simulink model "ai_optimal_path_v1"  (R2019a)
settings: Solver=FixedStepDiscrete  StartTime=0.0  StopTime=inf  FixedStep=0.2  RelTol=1e-3  EnableMultiTasking=on
undefined symbols (not defined in the file): Data, Data_SL_Info
libraries: robotlib x15
(part 1 of 2)
settings Model: Creator=USER  LastModifiedBy=USER
settings SolverCC: InsertRTBMode=Never (minimum delay)
settings DataIOCC: ReturnWorkspaceOutputs=off
settings OptimizationCC: StrengthReduction=on  PassReuseOutputArgsAs=Individual arguments  MaxStackSize=64  OptimizeBlockOrder=speed  OptimizationPriority=Speed  OptimizationCustomize=off  MultiThreadedLoops=on
settings DebuggingCC: ParameterTunabilityLossMsg=error  PregeneratedLibrarySubsystemCodeDiagnostic=none  ArithmeticOperatorsInVariantConditions=warning
settings HardwareCC: ProdBitPerPointer=32  ProdBitPerSizeT=32  ProdBitPerPtrDiffT=32  ProdLargestAtomicFloat=None  ProdIntDivRoundTo=Undefined  ProdEndianess=Unspecified  ProdWordSize=32  ProdHWDeviceType=Generic->Unspecified (assume 32-bit Generic)
settings SFSimCC: SimUseLocalCustomCode=off  MATLABDynamicMemAlloc=off
settings RTWCC: SystemTargetFile=ert.tlc  HardwareBoard=Robot Operating System (ROS)  TLCOptions="-aInlineSetEventsForThisBaseRateFcn=TLC_FALSE -aSuppressMultiTaskScheduler=TLC_FALSE  -aRateBasedStepFcn=0"  TemplateMakefile=ert_default_tmf  GenerateReport=on  RTWUseLocalCustomCode=off  Toolchain=Catkin  BuildConfiguration=Faster Runs  IncludeHyperlinkInReport=on  LaunchReport=on  TargetLang=C++  GenerateTraceInfo=on  GenerateTraceReport=on  GenerateTraceReportSl=on  GenerateTraceReportSf=on  GenerateTraceReportEml=on
settings CodeAppCC: ForceParamTrailComments=on  IgnoreCustomStorageClasses=off  OperatorAnnotations=on  SimulinkDataObjDesc=on  SFDataObjDesc=on  InsertBlockDesc=on
settings ERTTargetCC: SupportVariableSizeSignals=on

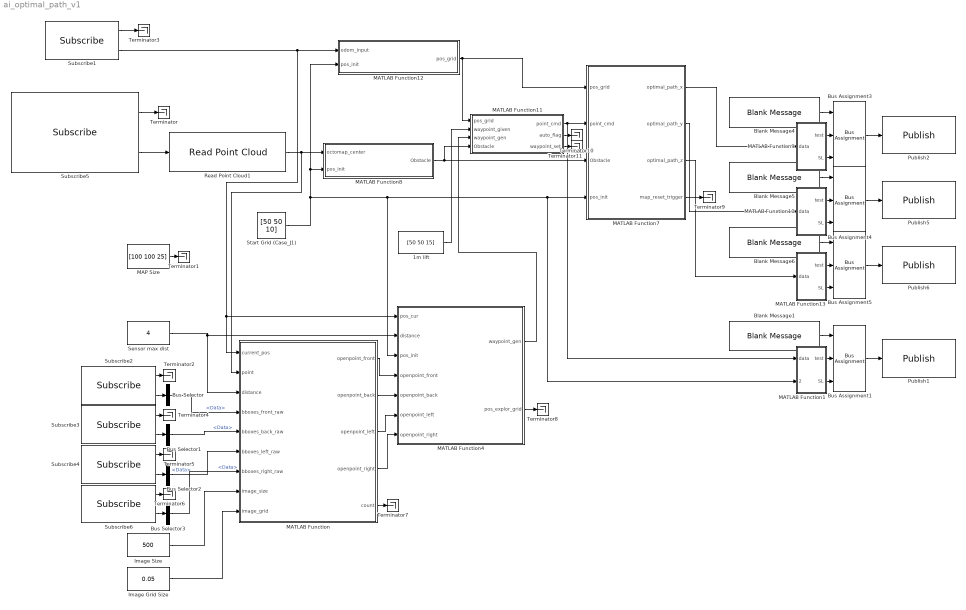
== system ai_optimal_path_v1 ==
  1m lift : Constant  Value=[50 50 15]
  Blank Message{1,4..6} (4 alike) : robotlib/Blank Message  messageClass=Message  entityType=std_msgs/Float32MultiArray  messageType=std_msgs/Float32MultiArray  SampleTime=-1
      settings: SourceProductBaseCode=RO
  Bus Assignment{1,3..5} (4 alike) : BusAssignment  AssignedSignals=Data,Data_SL_Info.CurrentLength
  Bus Selector{,1..3} (4 alike) : BusSelector  OutputSignals=Data
  Image Grid Size : Constant  Value=0.05
  Image Size : Constant  Value=500
  MAP Size : Constant  Value=[100 100 25]
  MATLAB Function : MATLAB Function  TreatAsAtomicUnit=on
  MATLAB Function1 : MATLAB Function  TreatAsAtomicUnit=on
  MATLAB Function10 : MATLAB Function  TreatAsAtomicUnit=on
  MATLAB Function11 : MATLAB Function  TreatAsAtomicUnit=on
  MATLAB Function12 : MATLAB Function  TreatAsAtomicUnit=on
  MATLAB Function13 : MATLAB Function  TreatAsAtomicUnit=on
  MATLAB Function4 : MATLAB Function  TreatAsAtomicUnit=on
  MATLAB Function7 : MATLAB Function  TreatAsAtomicUnit=on
  MATLAB Function8 : MATLAB Function  TreatAsAtomicUnit=on
  MATLAB Function9 : MATLAB Function  TreatAsAtomicUnit=on
  Publish1 : robotlib/Publish  topicSource=Specify your own  topic=/current_point_cmd  messageType=std_msgs/Float32MultiArray  messageQueueLength=1
      settings: SourceProductBaseCode=RO
  Publish2 : robotlib/Publish  topicSource=Specify your own  topic=/optimal_path_x  messageType=std_msgs/Float32MultiArray  messageQueueLength=1
      settings: SourceProductBaseCode=RO
  Publish5 : robotlib/Publish  topicSource=Specify your own  topic=/optimal_path_y  messageType=std_msgs/Float32MultiArray  messageQueueLength=1
      settings: SourceProductBaseCode=RO
  Publish6 : robotlib/Publish  topicSource=Specify your own  topic=/optimal_path_z  messageType=std_msgs/Float32MultiArray  messageQueueLength=1
      settings: SourceProductBaseCode=RO
  Read Point Cloud1 : robotlib/Read Point Cloud  MaximumPointCloudSize=[1, 650000]  PreserveStructure=off  ShowRGBOutput=off  ShowIntensityOutput=off  ShowErrorCodeOutput=off  VariableSizeOutputs=on
      settings: SourceProductName=Robotics System Toolbox  SourceProductBaseCode=RO
  Sensor max dist : Constant  Value=4
  Start Grid (Case_J1) : Constant  Value=[50 50 10]
  Subscribe1 : robotlib/Subscribe  topicSource=Select from ROS network  topic=/laser_odom_path  messageType=nav_msgs/Path  sampleTime=-1  messageQueueLength=1
      settings: SourceProductBaseCode=RO
  Subscribe2 : robotlib/Subscribe  topicSource=Select from ROS network  topic=/bboxes_front  messageType=std_msgs/Float32MultiArray  sampleTime=-1  messageQueueLength=1
      settings: SourceProductBaseCode=RO
  Subscribe3 : robotlib/Subscribe  topicSource=Select from ROS network  topic=/bboxes_back  messageType=std_msgs/Float32MultiArray  sampleTime=-1  messageQueueLength=1
      settings: SourceProductBaseCode=RO
  Subscribe4 : robotlib/Subscribe  topicSource=Select from ROS network  topic=/bboxes_left  messageType=std_msgs/Float32MultiArray  sampleTime=-1  messageQueueLength=1
      settings: SourceProductBaseCode=RO
  Subscribe5 : robotlib/Subscribe  topicSource=Select from ROS network  topic=/laser_cloud_map  messageType=sensor_msgs/PointCloud2  sampleTime=-1  messageQueueLength=1
      settings: SourceProductBaseCode=RO
  Subscribe6 : robotlib/Subscribe  topicSource=Select from ROS network  topic=/bboxes_right  messageType=std_msgs/Float32MultiArray  sampleTime=-1  messageQueueLength=1
      settings: SourceProductBaseCode=RO
  Terminator{,1..11} (12 alike) : Terminator
  wires:
  MATLAB Function9/1(test) -> Bus Assignment3/2
  Blank Message4/1 -> Bus Assignment3/1
  Bus Assignment4/1 -> Publish5/1
  Blank Message5/1 -> Bus Assignment4/1
  MATLAB Function9/2(SL) -> Bus Assignment3/3
  Subscribe1/1 -> Terminator3/1
  Subscribe1/2 -> MATLAB Function4/1(pos_cur), MATLAB Function/1(current_pos), MATLAB Function12/1(odom_input)
  MATLAB Function13/2(SL) -> Bus Assignment5/3
  Start Grid (Case_J1)/1 -> MATLAB Function4/3(pos_init), MATLAB Function1/2(pos_init), MATLAB Function7/4(pos_init), MATLAB Function8/2(pos_init), MATLAB Function12/2(pos_init)
  MATLAB Function12/1(pos_grid) -> MATLAB Function7/1(pos_grid), MATLAB Function11/1(pos_grid)
  MATLAB Function10/1(test) -> Bus Assignment4/2
  MATLAB Function13/1(test) -> Bus Assignment5/2
  Bus Assignment5/1 -> Publish6/1
  MATLAB Function10/2(SL) -> Bus Assignment4/3
  Blank Message6/1 -> Bus Assignment5/1
  Bus Assignment3/1 -> Publish2/1
  MAP Size/1 -> Terminator1/1
  MATLAB Function8/1(Obstacle) -> MATLAB Function11/4(Obstacle), MATLAB Function7/3(Obstacle)
  MATLAB Function7/1(optimal_path_x) -> MATLAB Function9/1(data)
  MATLAB Function7/2(optimal_path_y) -> MATLAB Function10/1(data)
  MATLAB Function7/3(optimal_path_z) -> MATLAB Function13/1(data)
  1m lift/1 -> MATLAB Function11/2(waypoint_given)
  Read Point Cloud1/1 -> MATLAB Function/2(point), MATLAB Function8/1(octomap_center)
  Subscribe5/2 -> Read Point Cloud1/1
  Subscribe5/1 -> Terminator/1
  MATLAB Function11/1(point_cmd) -> MATLAB Function7/2(point_cmd), MATLAB Function1/1(data)
  Subscribe2/1 -> Terminator2/1
  Subscribe3/1 -> Terminator4/1
  Subscribe4/1 -> Terminator5/1
  Subscribe6/1 -> Terminator6/1
  Subscribe2/2 -> Bus Selector/1
  Subscribe3/2 -> Bus Selector1/1
  Subscribe4/2 -> Bus Selector2/1
  Subscribe6/2 -> Bus Selector3/1
  Image Size/1 -> MATLAB Function/8(image_size)
  Image Grid Size/1 -> MATLAB Function/9(image_grid)
  Sensor max dist/1 -> MATLAB Function4/2(distance), MATLAB Function/3(distance)
  MATLAB Function/1(openpoint_front) -> MATLAB Function4/4(openpoint_front)
  MATLAB Function/2(openpoint_back) -> MATLAB Function4/5(openpoint_back)
  MATLAB Function/3(openpoint_left) -> MATLAB Function4/6(openpoint_left)
  MATLAB Function/4(openpoint_right) -> MATLAB Function4/7(openpoint_right)
  MATLAB Function/5(count) -> Terminator7/1
  MATLAB Function4/2(pos_explor_grid) -> Terminator8/1
  Bus Selector/1 -> MATLAB Function/4(bboxes_front_raw)  "<Data>"
  Bus Selector1/1 -> MATLAB Function/5(bboxes_back_raw)  "<Data>"
  Bus Selector2/1 -> MATLAB Function/6(bboxes_left_raw)  "<Data>"
  Bus Selector3/1 -> MATLAB Function/7(bboxes_right_raw)  "<Data>"
  MATLAB Function7/4(map_reset_trigger) -> Terminator9/1
  MATLAB Function4/1(waypoint_gen) -> MATLAB Function11/3(waypoint_gen)
  MATLAB Function11/2(auto_flag) -> Terminator10/1
  MATLAB Function11/3(waypoint_set) -> Terminator11/1
  MATLAB Function1/1(test) -> Bus Assignment1/2
  Bus Assignment1/1 -> Publish1/1
  MATLAB Function1/2(SL) -> Bus Assignment1/3
  Blank Message1/1 -> Bus Assignment1/1

== matlab function ai_optimal_path_v1/MATLAB Function1 ==
  data: data input size=[1 3]; test output size=[1 128]; SL output; pos_init input
function [test,SL]   = func(data,pos_init)

% test = single(nan(1,128));

test = single([data-pos_init', nan(1,125)]);
% for i = 1:length(data)
%     test(i) = single(data(i));
% end

SL = uint32(length(data));


end

== matlab function ai_optimal_path_v1/MATLAB Function ==
  data: current_pos input; point input; distance input; bboxes_front_raw input; bboxes_back_raw input; bboxes_left_raw input; bboxes_right_raw input; openpoint_front output; image_size input; image_grid input; openpoint_back output; openpoint_left output; openpoint_right output; count output
function [openpoint_front,openpoint_back,openpoint_left,openpoint_right,count] = fcn(current_pos,point,distance,bboxes_front_raw,bboxes_back_raw,bboxes_left_raw,bboxes_right_raw,image_size,image_grid)
% function [distance_ref_front,distance_ref_back,distance_ref_left,distance_ref_right] = fcn(point,I_front_rgb,I_back_rgb,I_left_rgb,I_right_rgb,bboxes_front_raw,bboxes_back_raw,bboxes_left_raw,bboxes_right_raw)
% image_grid = 0.05;

% pos_x = current_pos(1);
% pos_y = current_pos(2);
% pos_z = current_pos(3);
pos_x = current_pos.Poses(end).Pose.Position.X;
pos_y = current_pos.Poses(end).Pose.Position.Y;
pos_z = current_pos.Poses(end).Pose.Position.Z;

% image_size = 500;
% image_size = I_front_rgb(:,:,1);
% image_size = I_back_rgb(:,:,1);
% image_size = I_left_rgb(:,:,1);
% image_size = I_right_rgb(:,:,1);

openpoint_front = nan(5,6);
openpoint_back = nan(5,6);
openpoint_left = nan(5,6);
openpoint_right = nan(5,6);
count = zeros(5,4);
thickness = distance/2;
% thickness = 2;

% bboxes_front = int16(bboxes_front_raw);
% bboxes_back = int16(bboxes_back_raw);
% bboxes_left = int16(bboxes_left_raw);
% bboxes_right = int16(bboxes_right_raw);
bboxes_front = reshape(int16(bboxes_front_raw),[5, 4]);
bboxes_back = reshape(int16(bboxes_back_raw),[5, 4]);
bboxes_left = reshape(int16(bboxes_left_raw),[5, 4]);
bboxes_right = reshape(int16(bboxes_right_raw),[5, 4]);
% distance_ref_front=[];
% distance_ref_back=[];
% distance_ref_left=[];
% distance_ref_right=[];

distance_ref_front=nan(5,1);
distance_ref_back=nan(5,1);
distance_ref_left=nan(5,1);
distance_ref_right=nan(5,1);

% aaa=1;
% if ~isempty(bboxes_front)
if ~sum(bboxes_front)==0
    for aaa = 1:numel(nonzeros(bboxes_front))/4
        if (bboxes_front(aaa,1)+bboxes_front(aaa,3)/2) >= (image_size)/2
            distance_ref_front(aaa) = bboxes_front(aaa,1)+bboxes_front(aaa,3);
        else
            distance_ref_front(aaa) = bboxes_front(aaa,1);
        end
    end
    distance_ref_front= -(distance_ref_front - (image_size)/2)*image_grid;           % 醫뚰몴媛?(m)
end

% if ~isempty(bboxes_back)
if ~sum(bboxes_back)==0
    for aaa = 1:numel(nonzeros(bboxes_back))/4
        if (bboxes_back(aaa,1)+bboxes_back(aaa,3)/2) >= (image_size)/2
            distance_ref_back(aaa) = bboxes_back(aaa,1)+bboxes_back(aaa,3);
        else
            distance_ref_back(aaa) = bboxes_back(aaa,1);
        end
    end
    distance_ref_back= -(distance_ref_back - (image_size)/2)*image_grid;              % 醫뚰몴媛?(m)
end

% if ~isempty(bboxes_left)
if ~sum(bboxes_left)==0
    for aaa = 1:numel(nonzeros(bboxes_left))/4
        if (bboxes_left(aaa,1)+bboxes_left(aaa,3)/2) >= (image_size)/2
            distance_ref_left(aaa) = bboxes_left(aaa,1)+bboxes_left(aaa,3);
        else
            distance_ref_left(aaa) = bboxes_left(aaa,1);
        end
    end
    distance_ref_left= (distance_ref_left - (image_size)/2)*image_grid;              % 醫뚰몴媛?(m)
end

% if ~isempty(bboxes_right)
if ~sum(bboxes_right)==0
    for aaa = 1:numel(nonzeros(bboxes_right))/4
        if (bboxes_right(aaa,1)+bboxes_right(aaa,3)/2) >= (image_size)/2
            distance_ref_right(aaa) = bboxes_right(aaa,1)+bboxes_right(aaa,3);
        else
            distance_ref_right(aaa) = bboxes_right(aaa,1);
        end
    end
    distance_ref_right= (distance_ref_right - (image_size)/2)*image_grid;            % 醫뚰몴媛?(m)
end

% scale = 5;
scale = 10;
distance_fb_max=-ones(length(distance_ref_front),1)*image_grid*(image_size)/2;
distance_fb_min=ones(length(distance_ref_back),1)*image_grid*(image_size)/2;
distance_lr_max=-ones(length(distance_ref_left),1)*image_grid*(image_size)/2;
distance_lr_min=ones(length(distance_ref_right),1)*image_grid*(image_size)/2;

% distance_fb_max=ones(5,1)*distance;
% distance_fb_min=-ones(5,1)*distance;
% distance_lr_max=ones(5,1)*distance;
% distance_lr_min=-ones(5,1)*distance;
    
for bbb=1:length(point)
    %     if ~isempty(distance_ref_front)
    for aaa = 1:length(distance_ref_front)
        if ~isnan(distance_ref_front(aaa))
            if point(bbb,2)>=(distance_ref_front(aaa)-image_grid*scale) && point(bbb,2)<=(distance_ref_front(aaa)+image_grid*scale)
                if point(bbb,1) > distance_fb_max(aaa)
                    distance_fb_max(aaa) = point(bbb,1);
                end
            end
        end
    end
    %     if ~isempty(distance_ref_back)
    for aaa = 1:length(distance_ref_back)
        if ~isnan(distance_ref_back(aaa))
            if point(bbb,2)>=(distance_ref_back(aaa)-image_grid*scale) && point(bbb,2)<=(distance_ref_back(aaa)+image_grid*scale)
                if point(bbb,1) < distance_fb_min(aaa)
                    distance_fb_min(aaa) = point(bbb,1);
                end
            end
        end
    end
    %     if ~isempty(distance_ref_left)
    for aaa = 1:length(distance_ref_left)
        if ~isnan(distance_ref_left(aaa))
            if point(bbb,1)>=(distance_ref_left(aaa)-image_grid*scale) && point(bbb,1)<=(distance_ref_left(aaa)+image_grid*scale)
                if point(bbb,2) > distance_lr_max(aaa)
                    distance_lr_max(aaa) = point(bbb,2);
                end
            end
        end
    end
    %     if ~isempty(distance_ref_right)
    for aaa = 1:length(distance_ref_right)
        if ~isnan(distance_ref_right(aaa))
            if point(bbb,1)>=(distance_ref_right(aaa)-image_grid*scale) && point(bbb,1)<=(distance_ref_right(aaa)+image_grid*scale)
                if point(bbb,2) < distance_lr_min(aaa)
                    distance_lr_min(aaa) = point(bbb,2);
                end
            end
        end
    end
end
bboxes_transformed_front = -(double(bboxes_front)-[ones(5,1)*(image_size)/2, ones(5,1)*(image_size)/2, zeros(5,1), zeros(5,1)])*image_grid;
bboxes_transformed_back = -(double(bboxes_back)-[ones(5,1)*(image_size)/2, ones(5,1)*(image_size)/2, zeros(5,1), zeros(5,1)])*image_grid;
bboxes_transformed_left = (double(bboxes_left)-[ones(5,1)*(image_size)/2, ones(5,1)*(image_size)/2, zeros(5,1), zeros(5,1)]).*[ones(5,1), -ones(5,1), ones(5,1), -ones(5,1)]*image_grid;
bboxes_transformed_right = (double(bboxes_right)-[ones(5,1)*(image_size)/2, ones(5,1)*(image_size)/2, zeros(5,1), zeros(5,1)]).*[ones(5,1), -ones(5,1), ones(5,1), -ones(5,1)]*image_grid;

%(x,y,z,length,width,height)
% openpoint_front = [distance_fb_max-thickness/2,bboxes_transformed_front(:,1)+bboxes_transformed_front(:,3)/2,bboxes_transformed_front(:,2)+bboxes_transformed_front(:,4)/2,thickness*ones(length(distance_fb_max),1),abs(bboxes_transformed_front(:,3)),abs(bboxes_transformed_front(:,4))];                      
% openpoint_back = [distance_fb_min+thickness/2,bboxes_transformed_back(:,1)+bboxes_transformed_back(:,3)/2,bboxes_transformed_back(:,2)+bboxes_transformed_back(:,4)/2,thickness*ones(length(distance_fb_min),1),abs(bboxes_transformed_back(:,3)),abs(bboxes_transformed_back(:,4))];
% openpoint_left = [bboxes_transformed_left(:,1)+bboxes_transformed_left(:,3)/2 , distance_lr_max-thickness/2 , bboxes_transformed_left(:,2)+bboxes_transformed_left(:,4)/2,abs(bboxes_transformed_left(:,3)),thickness*ones(length(distance_lr_max),1),abs(bboxes_transformed_left(:,4))];
% openpoint_right = [bboxes_transformed_right(:,1)+bboxes_transformed_right(:,3)/2 , distance_lr_min+thickness/2 , bboxes_transformed_right(:,2)+bboxes_transformed_right(:,4)/2,abs(bboxes_transformed_right(:,3)),thickness*ones(length(distance_lr_min),1),abs(bboxes_transformed_right(:,4))];

for aaa = 1 : 5
    if ~(distance_fb_max(aaa) == -image_grid*(image_size)/2)
        openpoint_front(aaa,:) = [distance_fb_max(aaa)-thickness/2 , bboxes_transformed_front(aaa,1)+bboxes_transformed_front(aaa,3)/2+pos_y , bboxes_transformed_front(aaa,2)+bboxes_transformed_front(aaa,4)/2+pos_z , thickness , abs(bboxes_transformed_front(aaa,3)) , abs(bboxes_transformed_front(aaa,4))];
%         openpoint_front(aaa,:) = [distance_fb_max(aaa)-thickness/2+pos_x , bboxes_transformed_front(aaa,1)+bboxes_transformed_front(aaa,3)/2+pos_y , bboxes_transformed_front(aaa,2)+bboxes_transformed_front(aaa,4)/2+pos_z , thickness , abs(bboxes_transformed_front(aaa,3)) , abs(bboxes_transformed_front(aaa,4))];
    end
    if ~(distance_fb_min(aaa) == image_grid*(image_size)/2)
        openpoint_back(aaa,:) = [distance_fb_min(aaa)+thickness/2 , bboxes_transformed_back(aaa,1)+bboxes_transformed_back(aaa,3)/2+pos_y , bboxes_transformed_back(aaa,2)+bboxes_transformed_back(aaa,4)/2+pos_z , thickness , abs(bboxes_transformed_back(aaa,3)) , abs(bboxes_transformed_back(aaa,4))];
%         openpoint_back(aaa,:) = [distance_fb_min(aaa)+thickness/2+pos_x , bboxes_transformed_back(aaa,1)+bboxes_transformed_back(aaa,3)/2+pos_y , bboxes_transformed_back(aaa,2)+bboxes_transformed_back(aaa,4)/2+pos_z , thickness , abs(bboxes_transformed_back(aaa,3)) , abs(bboxes_transformed_back(aaa,4))];
    end
    if ~(distance_lr_max(aaa) == -image_grid*(image_size)/2)
        openpoint_left(aaa,:) = [bboxes_transformed_left(aaa,1)+bboxes_transformed_left(aaa,3)/2+pos_x , distance_lr_max(aaa)-thickness/2 , bboxes_transformed_left(aaa,2)+bboxes_transformed_left(aaa,4)/2+pos_z , abs(bboxes_transformed_left(aaa,3)) , thickness , abs(bboxes_transformed_left(aaa,4))];
%         openpoint_left(aaa,:) = [bboxes_transformed_left(aaa,1)+bboxes_transformed_left(aaa,3)/2+pos_x , distance_lr_max(aaa)-thickness/2+pos_y , bboxes_transformed_left(aaa,2)+bboxes_transformed_left(aaa,4)/2+pos_z , abs(bboxes_transformed_left(aaa,3)) , thickness , abs(bboxes_transformed_left(aaa,4))];
    end
    if ~(distance_lr_min(aaa) == image_grid*(image_size)/2)
        openpoint_right(aaa,:) = [bboxes_transformed_right(aaa,1)+bboxes_transformed_right(aaa,3)/2+pos_x , distance_lr_min(aaa)+thickness/2 , bboxes_transformed_right(aaa,2)+bboxes_transformed_right(aaa,4)/2+pos_z , abs(bboxes_transformed_right(aaa,3)) , thickness , abs(bboxes_transformed_right(aaa,4))];
%         openpoint_right(aaa,:) = [bboxes_transformed_right(aaa,1)+bboxes_transformed_right(aaa,3)/2+pos_x , distance_lr_min(aaa)+thickness/2+pos_y , bboxes_transformed_right(aaa,2)+bboxes_transformed_right(aaa,4)/2+pos_z , abs(bboxes_transformed_right(aaa,3)) , thickness , abs(bboxes_transformed_right(aaa,4))];
    end
end

for aaa = 1:5
    count_front = 0;
    count_back = 0;
    count_left = 0;
    count_right = 0;
    obstacle_check_front = 0;
    obstacle_check_back = 0;
    obstacle_check_left = 0;
    obstacle_check_right = 0;
    for bbb = 1:length(point)
        if ((point(bbb,1) > openpoint_front(aaa,1)-thickness/10) && (point(bbb,1) < openpoint_front(aaa,1)+thickness/10)) && (point(bbb,2) > openpoint_front(aaa,2)-thickness/10) && (point(bbb,2) < openpoint_front(aaa,2)+thickness/10)
%         if ((point(bbb,1) > openpoint_front(aaa,1)-thickness/2-thickness/10) && (point(bbb,1) < openpoint_front(aaa,1)-thickness/2+thickness/10)) && (point(bbb,2) > openpoint_front(aaa,2)-thickness/10) && (point(bbb,2) < openpoint_front(aaa,2)+thickness/10)
            count_front = count_front+1;
        end
        if ((point(bbb,1) > openpoint_back(aaa,1)-thickness/10) && (point(bbb,1) < openpoint_back(aaa,1)+thickness/10)) && (point(bbb,2) > openpoint_back(aaa,2)-thickness/10) && (point(bbb,2) < openpoint_back(aaa,2)+thickness/10)
%         if ((point(bbb,1) > openpoint_back(aaa,1)+thickness/2-thickness/10) && (point(bbb,1) < openpoint_back(aaa,1)+thickness/2+thickness/10)) && (point(bbb,2) > openpoint_back(aaa,2)-thickness/10) && (point(bbb,2) < openpoint_back(aaa,2)+thickness/10)
            count_back = count_back+1;
        end
        if ((point(bbb,1) > openpoint_left(aaa,1)-thickness/10) && (point(bbb,1) < openpoint_left(aaa,1)+thickness/10)) && (point(bbb,2) > openpoint_left(aaa,2)-thickness/10) && (point(bbb,2) < openpoint_left(aaa,2)+thickness/10)
%         if ((point(bbb,1) > openpoint_left(aaa,1)-thickness/10) && (point(bbb,1) < openpoint_left(aaa,1)+thickness/10)) && (point(bbb,2) > openpoint_left(aaa,2)-thickness/2-thickness/10) && (point(bbb,2) < openpoint_left(aaa,2)-thickness/2+thickness/10)
            count_left = count_left+1;
        end
        if ((point(bbb,1) > openpoint_right(aaa,1)-thickness/10) && (point(bbb,1) < openpoint_right(aaa,1)+thickness/10)) && (point(bbb,2) > openpoint_right(aaa,2)-thickness/10) && (point(bbb,2) < openpoint_right(aaa,2)+thickness/10)
%         if ((point(bbb,1) > openpoint_right(aaa,1)-thickness/10) && (point(bbb,1) < openpoint_right(aaa,1)+thickness/10)) && (point(bbb,2) > openpoint_right(aaa,2)+thickness/2-thickness/10) && (point(bbb,2) < openpoint_right(aaa,2)+thickness/2+thickness/10)
            count_right= count_right+1;
        end
        
        if ((point(bbb,1) > openpoint_front(aaa,1)-1) && (point(bbb,1) < openpoint_front(aaa,1)+1)) && ((point(bbb,2) > openpoint_front(aaa,2)-1) && (point(bbb,2) < openpoint_front(aaa,2)+1)) && ((point(bbb,3) > openpoint_front(aaa,3)-0.5) && (point(bbb,3) < openpoint_front(aaa,3)+0.5))
            obstacle_check_front = obstacle_check_front+1;
        end
        if ((point(bbb,1) > openpoint_back(aaa,1)-1) && (point(bbb,1) < openpoint_back(aaa,1)+1)) && ((point(bbb,2) > openpoint_back(aaa,2)-1) && (point(bbb,2) < openpoint_back(aaa,2)+1)) && ((point(bbb,3) > openpoint_back(aaa,3)-0.5) && (point(bbb,3) < openpoint_back(aaa,3)+0.5))
            obstacle_check_back = obstacle_check_back+1;
        end
        if ((point(bbb,1) > openpoint_left(aaa,1)-1) && (point(bbb,1) < openpoint_left(aaa,1)+1)) && ((point(bbb,2) > openpoint_left(aaa,2)-1) && (point(bbb,2) < openpoint_left(aaa,2)+1)) && ((point(bbb,3) > openpoint_left(aaa,3)-0.5) && (point(bbb,3) < openpoint_left(aaa,3)+0.5))
            obstacle_check_left = obstacle_check_left+1;
        end
        if ((point(bbb,1) > openpoint_right(aaa,1)-1) && (point(bbb,1) < openpoint_right(aaa,1)+1)) && ((point(bbb,2) > openpoint_right(aaa,2)-1) && (point(bbb,2) < openpoint_right(aaa,2)+1)) && ((point(bbb,3) > openpoint_right(aaa,3)-0.5) && (point(bbb,3) < openpoint_right(aaa,3)+0.5))
            obstacle_check_right= obstacle_check_right+1;
        end
        
    end
    %유효성 체크
    count(aaa,:) = [count_front, count_back, count_left, count_right];
    if count_front < 2 || obstacle_check_front > 0
%     if obstacle_check_front > 0
        openpoint_front(aaa,:) = nan(1,6);
    end
    if count_back< 2 || obstacle_check_back > 0
%     if obstacle_check_back > 0
        openpoint_back(aaa,:) = nan(1,6);
    end
    if count_left< 2 || obstacle_check_left > 0
%     if obstacle_check_left > 0
        openpoint_left(aaa,:) = nan(1,6);
    end
    if count_right< 2 || obstacle_check_right > 0
%     if obstacle_check_right > 0
        openpoint_right(aaa,:) = nan(1,6);
    end
end

== matlab function ai_optimal_path_v1/MATLAB Function4 ==
  data: pos_cur input; distance input; waypoint_gen output; pos_init input; openpoint_front input; openpoint_back input; openpoint_left input; openpoint_right input; pos_explor_grid output
function [waypoint_gen,pos_explor_grid] = fcn(pos_cur,distance,pos_init,openpoint_front,openpoint_back,openpoint_left,openpoint_right)

persistent explor_grid

if isempty(explor_grid)
    explor_grid = zeros(50,50,10);
end

% pos_x = current_pos(1);
% pos_y = current_pos(2);
% pos_z = current_pos(3);
pos_x = pos_cur.Poses(end).Pose.Position.X;
pos_y = pos_cur.Poses(end).Pose.Position.Y;
pos_z = pos_cur.Poses(end).Pose.Position.Z;

% grid_explor_size = 4;
grid_explor_size = distance/2;
grid_size = 0.2;
explor_map_init = [25, 25, 5];
pos_explor_grid = int32([pos_x/grid_explor_size+explor_map_init(1), pos_y/grid_explor_size+explor_map_init(2) , pos_z/grid_explor_size+explor_map_init(3)]);

explor_grid(pos_explor_grid(1),pos_explor_grid(2),pos_explor_grid(3))=1;



for abc=1:numel(openpoint_front)/6
    if ~isnan(openpoint_front(abc,1)) && ~isnan(openpoint_front(abc,2)) && ~isnan(openpoint_front(abc,3))
        if explor_grid(int16(openpoint_front(abc,1)/grid_explor_size+explor_map_init(1)),int16(openpoint_front(abc,2)/grid_explor_size+explor_map_init(2)),int16(openpoint_front(abc,3)/grid_explor_size+explor_map_init(3))) == 1
            openpoint_front(abc,:) = nan(1,6);
        end
    end
end
for abc=1:numel(openpoint_back)/6
    if ~isnan(openpoint_back(abc,1)) && ~isnan(openpoint_back(abc,2)) && ~isnan(openpoint_back(abc,3))
        if explor_grid(int16(openpoint_back(abc,1)/grid_explor_size+explor_map_init(1)),int16(openpoint_back(abc,2)/grid_explor_size+explor_map_init(2)),int16(openpoint_back(abc,3)/grid_explor_size+explor_map_init(3))) == 1
            openpoint_back(abc,:) = nan(1,6);
        end
    end
end
for abc=1:numel(openpoint_left)/6
    if ~isnan(openpoint_left(abc,1)) && ~isnan(openpoint_left(abc,2)) && ~isnan(openpoint_left(abc,3))
        if explor_grid(int16(openpoint_left(abc,1)/grid_explor_size+explor_map_init(1)),int16(openpoint_left(abc,2)/grid_explor_size+explor_map_init(2)),int16(openpoint_left(abc,3)/grid_explor_size+explor_map_init(3))) == 1
            openpoint_left(abc,:) = nan(1,6);
        end
    end
end
for abc=1:numel(openpoint_right)/6
    if ~isnan(openpoint_right(abc,1)) && ~isnan(openpoint_right(abc,2)) && ~isnan(openpoint_right(abc,3))
        if explor_grid(int16(openpoint_right(abc,1)/grid_explor_size+explor_map_init(1)),int16(openpoint_right(abc,2)/grid_explor_size+explor_map_init(2)),int16(openpoint_right(abc,3)/grid_explor_size+explor_map_init(3))) == 1
            openpoint_right(abc,:) = nan(1,6);
        end
    end
end



openpoint_front_grid = int16(openpoint_front/grid_size);
openpoint_back_grid = int16(openpoint_back/grid_size);
openpoint_left_grid = int16(openpoint_left/grid_size);
openpoint_right_grid = int16(openpoint_right/grid_size);



waypoint_gen_front = nan(5,3);
waypoint_gen_back = nan(5,3);
waypoint_gen_left = nan(5,3);
waypoint_gen_right = nan(5,3);

for aaa = 1:5
    if ~isnan(openpoint_front(aaa,1))
        waypoint_gen_front(aaa,:) = [openpoint_front_grid(aaa,1)+int16(pos_init(1)), openpoint_front_grid(aaa,2)+int16(pos_init(2)), openpoint_front_grid(aaa,3)+int16(pos_init(3))];
    end
    if ~isnan(openpoint_back(aaa,1))
        waypoint_gen_back(aaa,:) = [openpoint_back_grid(aaa,1)+int16(pos_init(1)), openpoint_back_grid(aaa,2)+int16(pos_init(2)), openpoint_back_grid(aaa,3)+int16(pos_init(3))];
    end
    if ~isnan(openpoint_left(aaa,1))
        waypoint_gen_left(aaa,:) = [openpoint_left_grid(aaa,1)+int16(pos_init(1)), openpoint_left_grid(aaa,2)+int16(pos_init(2)), openpoint_left_grid(aaa,3)+int16(pos_init(3))];
    end
    if ~isnan(openpoint_right(aaa,1))
        waypoint_gen_right(aaa,:) = [openpoint_right_grid(aaa,1)+int16(pos_init(1)), openpoint_right_grid(aaa,2)+int16(pos_init(2)), openpoint_right_grid(aaa,3)+int16(pos_init(3))];
    end
end

waypoint_gen = [waypoint_gen_front;waypoint_gen_back;waypoint_gen_left;waypoint_gen_right];

== matlab function ai_optimal_path_v1/MATLAB Function10 ==
  data: data input size=[128 1]; test output size=[1 128]; SL output
function [test,SL]   = func(data)

% test = single(nan(1,128));

test = data';
% for i = 1:length(data)
%     test(i) = single(data(i));
% end

SL = uint32(length(data));


end

== matlab function ai_optimal_path_v1/MATLAB Function11 ==
  data: pos_grid input; waypoint_given input; point_cmd output; waypoint_gen input; Obstacle input; auto_flag output; waypoint_set output
function [point_cmd,auto_flag,waypoint_set] = gen_waypoint(pos_grid,waypoint_given,waypoint_gen,Obstacle)

persistent flag autonomous_mode_flag waypoint_old waypoint_pre

if isempty(flag)
    flag = 1;
end
if isempty(autonomous_mode_flag)
    autonomous_mode_flag = 0;
end
if isempty(waypoint_old)
    waypoint_old = nan(20,3);
end
if isempty(waypoint_pre)
    waypoint_pre = nan(20,3);
    for aaa = 1:numel(waypoint_given)/3
        waypoint_pre(aaa,:)=waypoint_given(aaa,:);
    end
end
% if isempty(explor_grid)
%     explor_grid = zeros(30,20,6);
% end
% grid_explor_size = 1;
% explor_map_init = [15, 10, 3];
pos_grid = int32(pos_grid);
% pos_explor_grid = int32(pos_cur'./grid_explor_size+explor_map_size);
% pos_explor_grid = int32([pos_cur(1)/grid_explor_size+explor_map_init(1), pos_cur(2)/grid_explor_size+explor_map_init(2) , pos_cur(3)/grid_explor_size+explor_map_init(3)]);

% waypoint_gen_grid = waypoint_gen ./ 1 15,10,3;
% % 중복성 체크
% explor_grid(pos_explor_grid(1),pos_explor_grid(2),pos_explor_grid(3))=1;
% for abc=1:numel(waypoint_gen)/3
%     if ~isnan(waypoint_gen(abc,1)) && ~isnan(waypoint_gen(abc,2)) && ~isnan(waypoint_gen(abc,3))
%         if explor_grid(int32(waypoint_gen(abc,1)+explor_map_init(1)),int32(waypoint_gen(abc,2)+explor_map_init(2)),int32(waypoint_gen(abc,3)+explor_map_init(3))) == 1
%             waypoint_gen(abc,:) = nan(1,3);
%         end
%     end
% end


waypoint_pre_x = waypoint_pre(:,1);
waypoint_pre_y = waypoint_pre(:,2);
waypoint_pre_z = waypoint_pre(:,3);

point_cmd_temp = int32([waypoint_pre_x(flag) waypoint_pre_y(flag) waypoint_pre_z(flag)]);
waypoint_auto_set = nan(40,3);
waypoint_auto_set_sorted = nan(40,3);
waypoint_distance = nan(40,1);

for lll = 1:numel(waypoint_gen)/3
    if ~isnan(waypoint_gen(lll,1)) && ~isnan(waypoint_gen(lll,2)) && ~isnan(waypoint_gen(lll,3))
%         if waypoint_gen(lll,1)>0 && waypoint_gen(lll,2)>0 && waypoint_gen(lll,3)>0
            if Obstacle(waypoint_gen(lll,1),waypoint_gen(lll,2),waypoint_gen(lll,3)) == 1
                waypoint_gen(lll,:)=nan(1,3);
            end
%         end
    end
end


if autonomous_mode_flag==0
    if abs(point_cmd_temp(1)-pos_grid(1)) <= 0 && abs(point_cmd_temp(2)-pos_grid(2)) <= 0 && abs(point_cmd_temp(3)-pos_grid(3)) <= 0
        flag = flag + 1;
        
        if flag == numel(rmmissing(waypoint_pre))/3 + 1
            flag = numel(rmmissing(waypoint_pre))/3;
            autonomous_mode_flag = 1;
        end
    end
    
    % waypoint_gen_filtered = rmmissing(waypoint_gen);
    % if ~isempty(waypoint_gen_filtered)
    %     if flag == numel(waypoint_pre)/3
    %         waypoint_x = waypoint_gen_filtered(1,1);
    %         waypoint_y = waypoint_gen_filtered(1,2);
    %         waypoint_z = waypoint_gen_filtered(1,3);
    %     end
    % end
elseif autonomous_mode_flag==1
    waypoint_auto_old = rmmissing(waypoint_old);
    waypoint_auto_new = rmmissing(waypoint_gen);
    if isempty(waypoint_auto_old)
        waypoint_auto_old = waypoint_auto_new;
    end
    
    if ~isempty(waypoint_auto_old) && ~isempty(waypoint_auto_new)
        for mmm = numel(waypoint_auto_new)/3:-1:1
            changed_flag=0;
            for nnn = 1:numel(waypoint_auto_old)/3
                if ((waypoint_auto_new(mmm,1)-waypoint_auto_old(nnn,1))^2+(waypoint_auto_new(mmm,2)-waypoint_auto_old(nnn,2))^2+(waypoint_auto_new(mmm,3)-waypoint_auto_old(nnn,3))^2)<100
                    waypoint_auto_old(nnn,:)=waypoint_auto_new(mmm,:);
                    changed_flag=1;
                end
            end
            if changed_flag == 1
                waypoint_auto_new(mmm,:)=nan(1,3);
            end
        end
%         waypoint_auto_set_temp = cat(1,unique(waypoint_auto_old,'stable','rows'),waypoint_auto_new);

%             waypoint_auto_set_temp = rmmissing(cat(1,waypoint_auto_new,unique(waypoint_auto_old,'stable','rows')));
            waypoint_auto_set_temp = rmmissing(cat(1,unique(waypoint_auto_old,'stable','rows'),waypoint_auto_new));

        
        for aaa = 1:numel(waypoint_auto_set_temp)/3
            waypoint_auto_set(aaa,:)=waypoint_auto_set_temp(aaa,:);
            waypoint_distance(aaa) = (((waypoint_auto_set(aaa,1)-pos_grid(1))^2+(waypoint_auto_set(aaa,2)-pos_grid(2))^2+(waypoint_auto_set(aaa,3)-pos_grid(3))^2));
        end
        [~,waypoint_index]=sort(waypoint_distance);
        
        for aaa = 1:length(waypoint_index)
            waypoint_auto_set_sorted(aaa,:)=waypoint_auto_set(waypoint_index(aaa),:);
        end
%         waypoint_auto_set(1:aaa,:)=waypoint_auto_set_temp(waypoint_index,:);
        
        point_cmd_temp = int32([waypoint_auto_set_sorted(1,1), waypoint_auto_set_sorted(1,2), waypoint_auto_set_sorted(1,3)]);
        
        if abs(point_cmd_temp(1)-pos_grid(1)) <= 0 && abs(point_cmd_temp(2)-pos_grid(2)) <= 0 && abs(point_cmd_temp(3)-pos_grid(3)) <= 0
            waypoint_auto_set_sorted = [waypoint_auto_set_sorted(2:end,:); nan(1,3)];            
        end
        
        waypoint_old = waypoint_auto_set_sorted(1:20,:);
        
        
    else
        if ~isnan(waypoint_old(1,1)) && ~isnan(waypoint_old(1,2)) && ~isnan(waypoint_old(1,3))
            point_cmd_temp = int32([waypoint_old(1,1), waypoint_old(1,2), waypoint_old(1,3)]);
%             waypoint_pre = waypoint_old;
%             autonomous_mode_flag = 0;
%             flag = 1;

            if abs(point_cmd_temp(1)-pos_grid(1)) <= 0 && abs(point_cmd_temp(2)-pos_grid(2)) <= 0 && abs(point_cmd_temp(3)-pos_grid(3)) <= 0
                waypoint_old = [waypoint_old(2:end,:); nan(1,3)];            
            end


        else
            point_cmd_temp = int32([pos_grid(1), pos_grid(2), pos_grid(3)]);
        end
    end
end


% point_cmd = int32([waypoint_pre_x(flag) waypoint_pre_y(flag) waypoint_pre_z(flag)]);
point_cmd = point_cmd_temp;


auto_flag = autonomous_mode_flag;
waypoint_set = waypoint_auto_set_sorted;


end

== matlab function ai_optimal_path_v1/MATLAB Function12 ==
  data: odom_input input; pos_grid output; pos_init input
function pos_grid = odom_grid(odom_input,pos_init)

odom = zeros(1,3);


odom(1,1) = odom_input.Poses(end).Pose.Position.X;
odom(1,2) = odom_input.Poses(end).Pose.Position.Y;
odom(1,3) = odom_input.Poses(end).Pose.Position.Z;

start_point = [pos_init(1) pos_init(2) pos_init(3)];

% pos_x = int16(odom(1)/0.2+0.5);
% pos_y = int16(odom(2)/0.2+0.5);
% pos_z = int16(odom(3)/0.2+0.5);
pos_x = int16(odom(1)/0.2);
pos_y = int16(odom(2)/0.2);
pos_z = int16(odom(3)/0.2);

pos_grid = [pos_x+start_point(1) pos_y+start_point(2) pos_z+start_point(3)];


end

== matlab function ai_optimal_path_v1/MATLAB Function13 ==
  data: data input size=[128 1]; test output size=[1 128]; SL output
function [test,SL]   = func(data)


% test = single(nan(1,128));

test = data';
% for i = 1:length(data)
%     test(i) = single(data(i));
% end

SL = uint32(length(data));

end

== matlab function ai_optimal_path_v1/MATLAB Function7 ==
  data: pos_grid input; optimal_path_x output size=[128 1]; point_cmd input; Obstacle input; pos_init input; optimal_path_y output size=[128 1]; optimal_path_z output size=[128 1]; map_reset_trigger output
function [optimal_path_x,optimal_path_y,optimal_path_z,map_reset_trigger] = Astar_algorithm_function(pos_grid,point_cmd,Obstacle,pos_init)

    persistent optimal astar_restart curr_point hover_flag 

    if isempty(optimal)
        optimal = nan(128,3);
        hover_flag = 0;
        astar_restart = 1;
        curr_point = point_cmd;        
    end

    map_reset_trigger = 0;
    grid_size = 0.2;

    if (curr_point(1) ~= point_cmd(1)) || (curr_point(2) ~= point_cmd(2)) || (curr_point(3) ~= point_cmd(3))
        astar_restart = 1;
    end
    curr_point = point_cmd;
    
    if Obstacle(pos_grid(1), pos_grid(2), pos_grid(3)) == 1
        astar_restart = 0;
    end
    
    
%---------------------------------------------------------
% A* 시작
%---------------------------------------------------------
    if astar_restart == 1
        % ----------------------------------------------------- initilize
        astar_restart = 0;
        mapsize = [100 100 25];
        
        Height = mapsize(1);        % x
        Width = mapsize(2);         % y
        Alt = mapsize(3);            % z
        
        Start = pos_grid;
%         Goal = int32(point_cmd/grid_size + pos_init');          % 수정 
        Goal = int32(point_cmd);          % 수정 
        look = 2;
        H_weight = 1.3;
        
        G_cost = zeros(2*look+1,2*look+1,2*look+1);
        for i = 1:2*look+1
            for j = 1:2*look+1
                for k = 1:2*look+1
                    temp = [look+1 look+1 look+1]-[i j k];
                    G_cost(i,j,k) = (min(sqrt(sum(abs(temp).^2,2))));
                end
            end
        end
        
        G_top2 = G_cost(:,:,1);
        G_top1 = G_cost(:,:,2);
        G_mid = G_cost(:,:,3);
        G_bottom1 = G_cost(:,:,4);
        G_bottom2 = G_cost(:,:,5);
        
        
        GScore = inf(Height,Width,Alt);
        GScore_temp = zeros(2*look+1,2*look+1,2*look+1);
        HScore = zeros(Height,Width,Alt);
        FScore = inf(Height,Width,Alt);
        ClosedMAT = zeros(Height,Width,Alt);
        CX = int32(Start(1));
        CY = int32(Start(2));
        CZ = int32(Start(3));
        ParentX = inf(Height,Width,Alt);
        ParentY = inf(Height,Width,Alt);
        ParentZ = inf(Height,Width,Alt);
        ParentX(CX,CY,CZ) = CX;
        ParentY(CX,CY,CZ) = CY;
        ParentZ(CX,CY,CZ) = CZ;
        hover_flag = 0;
        
        %%%%%%%%%%%%%%%% Define Heuristic %%%%%%%%%%%%%%%%%%%%%%%
        for k=1:Alt
            for j=1:Width
                for i=1:Height
                    
                    temp = (int32(Goal) - int32([i j k])) ;
                    Distance=(min(sqrt(sum(abs(temp).^2,2))));
                    HScore(i,j,k)=Distance*H_weight;               % (1+sqrt(2))/sqrt(3)
                    
                end
            end
        end
        
        FScore(Start(1),Start(2),Start(3)) = HScore(Start(1),Start(2),Start(3));
        GScore(Start(1),Start(2),Start(3)) = 0;
        ClosedMAT(Obstacle==1)=1;
        REACHGOAL = 0;
        
        while 1
            fprintf("A* loop \n");
            MinFScore = min(min(min(FScore)));         % Find Minimun FScore
            
            if isinf(MinFScore)
                hover_flag = 1;
                astar_restart = 1;
                map_reset_trigger = 1;
                fprintf("No path -> restart A*, Map reset \n");
                break
            end
            
            [minF_x,minF_y] = find(FScore==MinFScore);
            HScore_temp = inf(1,10);
            
            minHScore = 1;
            for i = 1:length(minF_x)
                Current_pose_temp = [minF_x(i) rem(minF_y(i),Width) fix(minF_y(i)/Width)+1];     % H가 가장 적은걸로 먼저 선택
                CX_temp=Current_pose_temp(1);
                CY_temp=Current_pose_temp(2);
                CZ_temp=Current_pose_temp(3);
                HScore_temp(i) = HScore(CX_temp,CY_temp,CZ_temp);
                minHScore = find(HScore_temp == min(HScore_temp));
            end
            
            Current_pose = int32([minF_x(minHScore(1)) rem(minF_y(minHScore(1)),Width) fix(minF_y(minHScore(1))/Width)+1]);     % H가 가장 적은걸로 먼저 선택
            CX=Current_pose(1);
            CY=Current_pose(2);
            CZ=Current_pose(3);

            GScore_temp(:,:,1) = GScore(CX,CY,CZ) + G_top2;
            GScore_temp(:,:,2) = GScore(CX,CY,CZ) + G_top1;
            GScore_temp(:,:,3) = GScore(CX,CY,CZ) + G_mid;
            GScore_temp(:,:,4) = GScore(CX,CY,CZ) + G_bottom1;
            GScore_temp(:,:,5) = GScore(CX,CY,CZ) + G_bottom2;
            
            %%%%%%%%%%%%% GScore update %%%%%%%%%%%%%
            GScore(CX-look:CX+look,CY-look:CY+look,CZ+2) = min(GScore_temp(:,:,1),GScore(CX-look:CX+look,CY-look:CY+look,CZ+2)) ;
            GScore(CX-look:CX+look,CY-look:CY+look,CZ+1) = min(GScore_temp(:,:,2),GScore(CX-look:CX+look,CY-look:CY+look,CZ+1));
            GScore(CX-look:CX+look,CY-look:CY+look,CZ) = min(GScore_temp(:,:,3), GScore(CX-look:CX+look,CY-look:CY+look,CZ));
            GScore(CX-look:CX+look,CY-look:CY+look,CZ-1) = min(GScore_temp(:,:,4),GScore(CX-look:CX+look,CY-look:CY+look,CZ-1));
            GScore(CX-look:CX+look,CY-look:CY+look,CZ-2) = min(GScore_temp(:,:,5),GScore(CX-look:CX+look,CY-look:CY+look,CZ-2));
            
            FScore = GScore + HScore;
            ClosedMAT(CX-(look-1):CX+(look-1),CY-(look-1):CY+(look-1),CZ-(look-1):CZ+(look-1)) = 1;
            FScore(ClosedMAT==1) = inf;
            
            [G_row1,G_col1] = find( GScore(CX-look:CX+look,CY-look:CY+look,CZ+2) == GScore_temp(:,:,1) );
            [G_row2,G_col2] = find( GScore(CX-look:CX+look,CY-look:CY+look,CZ+1) == GScore_temp(:,:,2) );
            [G_row3,G_col3] = find( GScore(CX-look:CX+look,CY-look:CY+look,CZ) == GScore_temp(:,:,3) );
            [G_row4,G_col4] = find( GScore(CX-look:CX+look,CY-look:CY+look,CZ-1) == GScore_temp(:,:,4) );
            [G_row5,G_col5] = find( GScore(CX-look:CX+look,CY-look:CY+look,CZ-2) == GScore_temp(:,:,5) );
            
            G_row1 = int32(G_row1);
            G_row2 = int32(G_row2);
            G_row3 = int32(G_row3);
            G_row4 = int32(G_row4);
            G_row5 = int32(G_row5);
            
            G_col1 = int32(G_col1);
            G_col2 = int32(G_col2);
            G_col3 = int32(G_col3);
            G_col4 = int32(G_col4);
            G_col5 = int32(G_col5);
            
            G_row1 = G_row1+CX-(look+1);
            G_row2 = G_row2+CX-(look+1);
            G_row3 = G_row3+CX-(look+1);
            G_row4 = G_row4+CX-(look+1);
            G_row5 = G_row5+CX-(look+1);
            
            G_col1 = G_col1+CY-(look+1);
            G_col2 = G_col2+CY-(look+1);
            G_col3 = G_col3+CY-(look+1);
            G_col4 = G_col4+CY-(look+1);
            G_col5 = G_col5+CY-(look+1);
            
            for i = 1:length(G_row1)
                ParentX(G_row1(i),G_col1(i),CZ+2) = CX;
                ParentY(G_row1(i),G_col1(i),CZ+2) = CY;
                ParentZ(G_row1(i),G_col1(i),CZ+2) = CZ;
            end
            
            for i = 1:length(G_row2)
                ParentX(G_row2(i),G_col2(i),CZ+1) = CX;
                ParentY(G_row2(i),G_col2(i),CZ+1) = CY;
                ParentZ(G_row2(i),G_col2(i),CZ+1) = CZ;
            end
            
            for i = 1:length(G_row3)
                if G_row3(i)==CX && G_col3(i)==CY
                    continue
                end
                ParentX(G_row3(i),G_col3(i),CZ) = CX;
                ParentY(G_row3(i),G_col3(i),CZ) = CY;
                ParentZ(G_row3(i),G_col3(i),CZ) = CZ;
            end
            
            for i = 1:length(G_row4)
                ParentX(G_row4(i),G_col4(i),CZ-1) = CX;
                ParentY(G_row4(i),G_col4(i),CZ-1) = CY;
                ParentZ(G_row4(i),G_col4(i),CZ-1) = CZ;
            end
            
            for i = 1:length(G_row5)
                ParentX(G_row5(i),G_col5(i),CZ-2) = CX;
                ParentY(G_row5(i),G_col5(i),CZ-2) = CY;
                ParentZ(G_row5(i),G_col5(i),CZ-2) = CZ;
            end
            
            if abs(Goal(1)-CX)<=(look-1) && abs(Goal(2)-CY)<=(look-1) && abs(Goal(3)-CZ)<=(look-1)
                REACHGOAL = 1;
                fprintf("path founded\n");
                break
            end
        end
        
        optimal = nan(128,3);
        if REACHGOAL
            optimal(1,:) = [Goal(1) Goal(2) Goal(3)];
            k=2;
            while 1
                CX_temp = int32(ParentX(CX,CY,CZ));
                CY_temp = int32(ParentY(CX,CY,CZ));
                CZ_temp = int32(ParentZ(CX,CY,CZ));
                
                CX = CX_temp;
                CY = CY_temp;
                CZ = CZ_temp;
                
                optimal(k,:) = [CX CY CZ];
                k = k+1;
                
                if CX==Start(1) && CY==Start(2) && CZ==Start(3)
                    break
                end
            end
        end
        
    end
    
    if hover_flag == 0
            nan_check = isnan(optimal(:,1));
            for i = 1:1:128
                if nan_check(i) == 0
                    %fprintf("i:%d (%d,%d,%d) %d    ", int32(i), int32(optimal(i,1)), int32(optimal(i,2)), int32(optimal(i,3)), int32(Obstacle(optimal(i,1), optimal(i,2), optimal(i,3))));
                    if Obstacle(optimal(i,1), optimal(i,2), optimal(i,3)) == 1
                        astar_restart = 1;
                        fprintf("path collision! \n");
                        break;
                    end
                    %fprintf("not break \n");
                end
                astar_restart = 0;
            end
            % fprintf("collision check done \n");
    end
        
    if hover_flag == 1
        fprintf("hover flag on \n");
        hover_point = nan(128,3);
        hover_point(1,:) = [pos_grid(1) pos_grid(2) pos_grid(3)];
        optimal_path_x = flip(single( (hover_point(:,1)-pos_init(1)) * grid_size ));      % grid_size = 0.2,
        optimal_path_y = flip(single( (hover_point(:,2)-pos_init(2)) * grid_size ));
        optimal_path_z = flip(single( (hover_point(:,3)-pos_init(3)) * grid_size ));
    else
        optimal_path_x = flip(single( (optimal(:,1)-pos_init(1)) * grid_size ));      % grid_size = 0.2
        optimal_path_y = flip(single( (optimal(:,2)-pos_init(2)) * grid_size ));
        optimal_path_z = flip(single( (optimal(:,3)-pos_init(3)) * grid_size ));
    end
    
    
end
